simulink model "sampleModel1414"  (R2023a)
settings: Solver=VariableStepAuto  StartTime=0.0  StopTime=10.0  RelTol=1e-3
libraries: hdlsllib x2, simulink x2
settings Model: Creator=user1  LastModifiedBy=user1

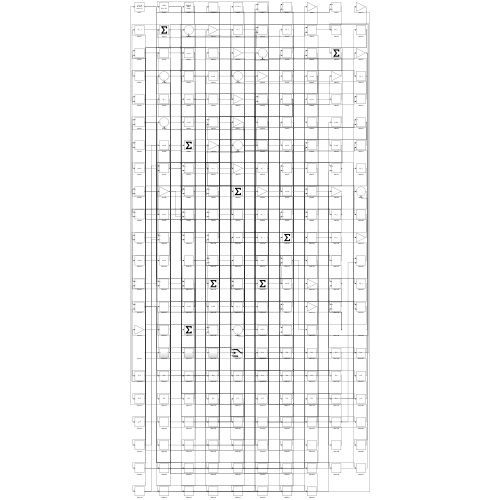
[thumbnail: Simulink's stored preview of the top-level diagram]
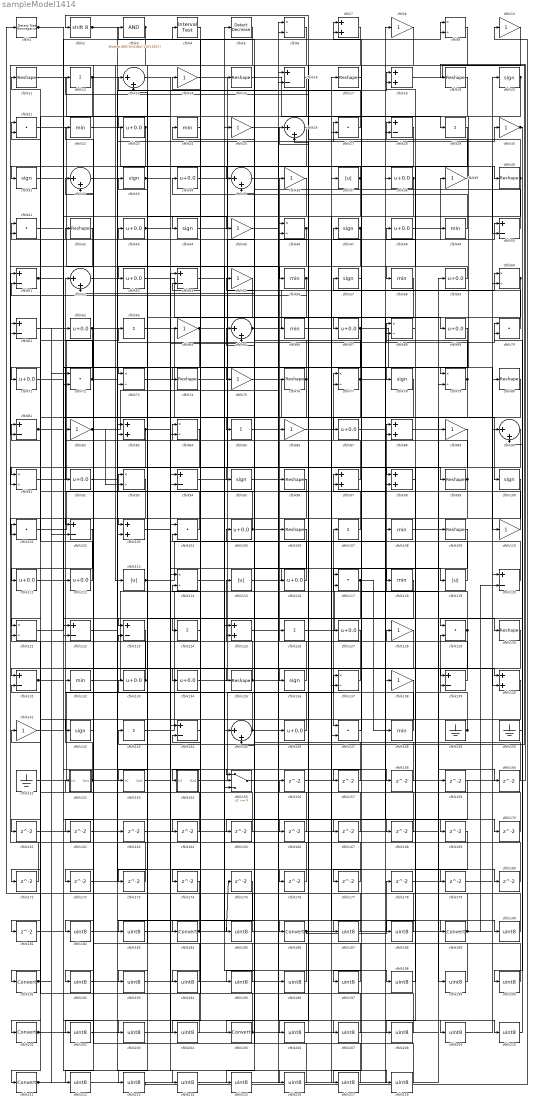
== system sampleModel1414 ==
  cfblk1 : hdlsllib/Logic and Bit Operations/Detect Rise Nonnegative  vinit=0  OutDataTypeStr=boolean
  cfblk{8,10,14,25,30,36,39,45,55,64,75,82,86,89,110,128,138,141} (18 alike) : Gain
  cfblk{20,31,33,44,47,57,78,95,100,136,142} (11 alike) : Signum
  cfblk{21,27,41,70,72,101,104,117,129,147} (10 alike) : DotProduct  OutDataTypeStr=Inherit: Inherit via internal rule
  cfblk{16,28,50..51,54,61,81,94,102,120,122..123,131,139,144} (15 alike) : Sum  Inputs=+-
  cfblk{7,18,83,88,97..98,103,125,140} (9 alike) : Sum
  cfblk{23,34,38,43,48,53,59,62,67,69,71,87,92,105,111..112,116,127,133..134,146} (21 alike) : Bias  Bias=0.0  SaturateOnIntegerOverflow=off
  cfblk{11,15,17,19,40,42,74,76,80,96,99,106,109,130,135} (15 alike) : Reshape
  cfblk{12,29,63,85,107,124,126,143} (8 alike) : Sum  Inputs=+
  cfblk{22,24,49,56,58,66,108,118,132,148} (10 alike) : MinMax
  cfblk{37,113,115,119} (4 alike) : Abs  SaturateOnIntegerOverflow=off
  cfblk{6,9,46,60,68,73,77,79,84,91,93,114,121,137} (14 alike) : Product  Inputs=*/  RndMeth=Zero  SaturateOnIntegerOverflow=on
  cfblk{13,26,32,35,52,65,90,145} (8 alike) : Sum  Inputs=|++
  cfblk149 : Ground
  cfblk150 : Ground
  cfblk151 : Ground
  cfblk152 : Subsystem
      settings: LibrarySourceBlock=|
      | hdlsllib/Ports &
      | Subsystems/Subsystem
  cfblk153 : Subsystem
      settings: LibrarySourceBlock=|
      | hdlsllib/Ports &
      | Subsystems/Subsystem
  cfblk154 : Subsystem
      settings: LibrarySourceBlock=|
      | hdlsllib/Ports &
      | Subsystems/Subsystem
  cfblk155 : Switch  SaturateOnIntegerOverflow=off  InputSameDT=off
  cfblk{156..181} (26 alike) : Delay  SampleTime=1
  cfblk{182..183,185,187..188,190,192..200,202..204,206..210,212..218} (30 alike) : DataTypeConversion  OutDataTypeStr=uint8  SaturateOnIntegerOverflow=off  RndMeth=Floor
  cfblk{184,186,189,191,201,205,211} (7 alike) : DataTypeConversion  SaturateOnIntegerOverflow=off  RndMeth=Floor
  cfblk2 : ArithShift  BitShiftNumber=8
  cfblk3 : simulink/Logic and Bit Operations/Bitwise Operator  logicop=AND  UseBitMask=on  BitMask=bin2dec('11011001')  BitMaskRealWorld=Stored Integer
      settings: LibrarySourceBlock=|
      | hdlsllib/Logic and Bit
      | Operations/Bitwise
      | Operator
  cfblk4 : hdlsllib/Logic and Bit Operations/Interval Test  IntervalClosedRight=on  uplimit=0.5  IntervalClosedLeft=on  lowlimit=-0.5  OutDataTypeStr=boolean
  cfblk5 : simulink/Logic and Bit Operations/Detect Decrease  vinit=0.0  OutDataTypeStr=boolean
      settings: LibrarySourceBlock=|
      | hdlsllib/Logic and Bit
      | Operations/Detect
      | Decrease
  wires:
  cfblk97/1 -> cfblk36/1
  cfblk57/1 -> cfblk103/1
  cfblk53/1 -> cfblk67/1
  cfblk3/1 -> cfblk113/1, cfblk81/2
  cfblk136/1 -> cfblk86/1
  cfblk39/1 -> cfblk2/1
  cfblk20/1 -> cfblk78/1, cfblk71/1
  cfblk145/1 -> cfblk33/1, cfblk49/1
  cfblk98/1 -> cfblk48/1
  cfblk50/1 -> cfblk24/1
  cfblk113/1 -> cfblk38/1, cfblk117/2
  cfblk152/1(Out1) -> cfblk52/1, cfblk155/2
  cfblk107/1 -> cfblk97/1
  cfblk89/1 -> cfblk211/1
  cfblk79/1 -> cfblk28/1, cfblk187/1
  cfblk94/1 -> cfblk60/1
  cfblk34/1 -> cfblk40/1
  cfblk30/1 -> cfblk129/1, cfblk200/1
  cfblk45/1 -> cfblk106/1
  cfblk134/1 -> cfblk50/1
  cfblk148/1 -> cfblk84/1
  cfblk135/1 -> cfblk115/1, cfblk210/1
  cfblk26/1 -> cfblk205/1
  cfblk77/1 -> cfblk41/1, cfblk127/1, cfblk140/1, cfblk161/1
  cfblk63/1 -> cfblk100/1
  cfblk14/1 -> cfblk99/1
  cfblk48/1 -> cfblk39/1
  cfblk124/1 -> cfblk14/1
  cfblk91/1 -> cfblk63/1
  cfblk44/1 -> cfblk27/1
  cfblk129/1 -> cfblk47/1, cfblk139/1
  cfblk76/1 -> cfblk3/1, cfblk103/2
  cfblk27/1 -> cfblk13/1
  cfblk60/1 -> cfblk98/2, cfblk204/1
  cfblk2/1 -> cfblk56/1, cfblk176/1
  cfblk123/1 -> cfblk131/1
  cfblk21/1 -> cfblk125/1
  cfblk149/1 -> cfblk129/2, cfblk68/2, cfblk139/2
  cfblk18/1 -> cfblk143/1
  cfblk151/1 -> cfblk15/1
  cfblk65/1 -> cfblk20/1, cfblk9/1
  cfblk62/1 -> cfblk92/1, cfblk30/1
  cfblk109/1 -> cfblk147/1
  cfblk22/1 -> cfblk50/2
  cfblk75/1 -> cfblk109/1
  cfblk35/1 -> cfblk69/1
  cfblk82/1 -> cfblk76/1, cfblk93/2
  cfblk81/1 -> cfblk122/1, cfblk140/2
  cfblk67/1 -> cfblk110/1, cfblk122/2
  cfblk70/1 -> cfblk7/1
  cfblk68/1 -> cfblk18/1
  cfblk143/1 -> cfblk107/1
  cfblk13/1 -> cfblk45/1
  cfblk133/1 -> cfblk101/1, cfblk93/1
  cfblk154/1(Out1) -> cfblk137/1
  cfblk99/1 -> cfblk22/1, cfblk77/2, cfblk165/1
  cfblk46/1 -> cfblk94/2, cfblk74/1
  cfblk11/1 -> cfblk84/2
  cfblk96/1 -> cfblk101/2
  cfblk132/1 -> cfblk59/1
  cfblk28/1 -> cfblk41/2
  cfblk117/1 -> cfblk153/1(In1), cfblk148/1
  cfblk155/1 -> cfblk19/1
  cfblk131/1 -> cfblk102/2, cfblk207/1, cfblk209/1
  cfblk1/1 -> cfblk44/1, cfblk9/2
  cfblk61/1 -> cfblk123/1
  cfblk150/1 -> cfblk70/1
  cfblk105/1 -> cfblk119/1, cfblk21/2
  cfblk85/1 -> cfblk126/1
  cfblk64/1 -> cfblk25/1, cfblk102/1
  cfblk38/1 -> cfblk95/1, cfblk87/1
  cfblk139/1 -> cfblk82/1
  cfblk115/1 -> cfblk117/1
  cfblk42/1 -> cfblk61/2
  cfblk9/1 -> cfblk35/1
  cfblk37/1 -> cfblk154/1(In1), cfblk31/1
  cfblk126/1 -> cfblk88/1
  cfblk54/1 -> cfblk145/1
  cfblk55/1 -> cfblk73/1
  cfblk49/1 -> cfblk34/1
  cfblk138/1 -> cfblk201/1
  cfblk114/1 -> cfblk186/1
  cfblk121/1 -> cfblk7/2
  cfblk59/1 -> cfblk53/1
  cfblk15/1 -> cfblk29/1
  cfblk12/1 -> cfblk72/2, cfblk180/1
  cfblk104/1 -> cfblk21/1
  cfblk146/1 -> cfblk42/1
  cfblk137/1 -> cfblk136/1
  cfblk29/1 -> cfblk58/1
  cfblk120/1 -> cfblk54/2
  cfblk25/1 -> cfblk116/1
  cfblk56/1 -> cfblk51/2, cfblk134/1
  cfblk147/1 -> cfblk57/1
  cfblk69/1 -> cfblk142/1
  cfblk73/1 -> cfblk146/1
  cfblk116/1 -> cfblk55/1
  cfblk119/1 -> cfblk46/2
  cfblk8/1 -> cfblk23/1
  cfblk4/1 -> cfblk184/1
  cfblk72/1 -> cfblk18/2, cfblk11/1, cfblk98/1
  cfblk40/1 -> cfblk137/2, cfblk12/1
  cfblk47/1 -> cfblk124/1, cfblk155/3, cfblk206/1
  cfblk112/1 -> cfblk81/1
  cfblk51/1 -> cfblk130/1, cfblk75/1, cfblk91/1
  cfblk71/1 -> cfblk112/1
  cfblk43/1 -> cfblk118/1, cfblk155/1
  cfblk86/1 -> cfblk77/1
  cfblk66/1 -> cfblk189/1
  cfblk58/1 -> cfblk135/1
  cfblk101/1 -> cfblk8/1
  cfblk31/1 -> cfblk85/1
  cfblk23/1 -> cfblk121/1, cfblk192/1
  cfblk103/1 -> cfblk70/2
  cfblk122/1 -> cfblk68/1
  cfblk33/1 -> cfblk79/1, cfblk179/1
  cfblk16/1 -> cfblk191/1
  cfblk110/1 -> cfblk97/2
  cfblk19/1 -> cfblk111/1
  cfblk80/1 -> cfblk83/2
  cfblk83/1 -> cfblk65/2, cfblk91/2
  cfblk156/1 -> cfblk27/2
  cfblk78/1 -> cfblk157/1
  cfblk157/1 -> cfblk104/1
  cfblk41/1 -> cfblk158/1
  cfblk158/1 -> cfblk94/1
  cfblk88/1 -> cfblk160/1
  cfblk160/1 -> cfblk52/2
  cfblk161/1 -> cfblk79/2
  cfblk140/1 -> cfblk162/1
  cfblk162/1 -> cfblk54/1
  cfblk92/1 -> cfblk163/1
  cfblk24/1 -> cfblk164/1
  cfblk164/1 -> cfblk123/2
  cfblk165/1 -> cfblk131/2
  cfblk7/1 -> cfblk166/1
  cfblk166/1 -> cfblk65/1
  cfblk111/1 -> cfblk167/1
  cfblk167/1 -> cfblk35/2
  cfblk95/1 -> cfblk168/1
  cfblk168/1 -> cfblk125/2
  cfblk87/1 -> cfblk169/1
  cfblk153/1(Out1) -> cfblk170/1
  cfblk170/1 -> cfblk145/2
  cfblk84/1 -> cfblk171/1
  cfblk171/1 -> cfblk61/1
  cfblk93/1 -> cfblk172/1
  cfblk172/1 -> cfblk73/2
  cfblk130/1 -> cfblk173/1
  cfblk173/1 -> cfblk51/1
  cfblk118/1 -> cfblk174/1
  cfblk174/1 -> cfblk1/1
  cfblk176/1 -> cfblk13/2
  cfblk17/1 -> cfblk177/1
  cfblk177/1 -> cfblk83/1
  cfblk178/1 -> cfblk120/1
  cfblk179/1 -> cfblk60/2
  cfblk180/1 -> cfblk46/1
  cfblk102/1 -> cfblk181/1
  cfblk5/1 -> cfblk182/1
  cfblk182/1 -> cfblk37/1
  cfblk36/1 -> cfblk183/1
  cfblk183/1 -> cfblk5/1
  cfblk184/1 -> cfblk175/1, cfblk43/1
  cfblk100/1 -> cfblk185/1
  cfblk185/1 -> cfblk4/1
  cfblk186/1 -> cfblk178/1, cfblk80/1
  cfblk187/1 -> cfblk114/1
  cfblk169/1 -> cfblk188/1
  cfblk188/1 -> cfblk114/2
  cfblk189/1 -> cfblk156/1, cfblk120/2
  cfblk52/1 -> cfblk190/1
  cfblk190/1 -> cfblk66/1
  cfblk191/1 -> cfblk121/2, cfblk72/1
  cfblk192/1 -> cfblk16/1
  cfblk175/1 -> cfblk193/1
  cfblk193/1 -> cfblk16/2
  cfblk144/1 -> cfblk194/1
  cfblk194/1 -> cfblk152/1(In1)
  cfblk159/1 -> cfblk195/1
  cfblk195/1 -> cfblk144/1
  cfblk125/1 -> cfblk196/1
  cfblk196/1 -> cfblk144/2
  cfblk128/1 -> cfblk197/1
  cfblk197/1 -> cfblk133/1
  cfblk74/1 -> cfblk198/1
  cfblk198/1 -> cfblk128/1
  cfblk108/1 -> cfblk199/1
  cfblk199/1 -> cfblk96/1
  cfblk200/1 -> cfblk108/1
  cfblk201/1 -> cfblk159/1, cfblk88/2
  cfblk127/1 -> cfblk202/1
  cfblk202/1 -> cfblk138/1
  cfblk141/1 -> cfblk203/1
  cfblk203/1 -> cfblk64/1
  cfblk204/1 -> cfblk141/1
  cfblk205/1 -> cfblk147/2, cfblk132/1
  cfblk206/1 -> cfblk26/1
  cfblk207/1 -> cfblk26/2
  cfblk90/1 -> cfblk208/1
  cfblk208/1 -> cfblk104/2
  cfblk209/1 -> cfblk90/1
  cfblk210/1 -> cfblk90/2
  cfblk211/1 -> cfblk28/2, cfblk17/1, cfblk62/1
  cfblk142/1 -> cfblk212/1
  cfblk212/1 -> cfblk89/1
  cfblk6/1 -> cfblk213/1
  cfblk213/1 -> cfblk10/1
  cfblk181/1 -> cfblk214/1
  cfblk214/1 -> cfblk6/1
  cfblk106/1 -> cfblk215/1
  cfblk215/1 -> cfblk6/2
  cfblk32/1 -> cfblk216/1
  cfblk216/1 -> cfblk105/1
  cfblk10/1 -> cfblk217/1
  cfblk217/1 -> cfblk32/1
  cfblk163/1 -> cfblk218/1
  cfblk218/1 -> cfblk32/2

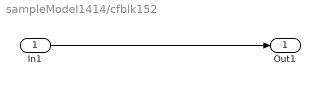
== system sampleModel1414/cfblk152 ==
  In1 : Inport
  Out1 : Outport
  wires:
  In1/1 -> Out1/1

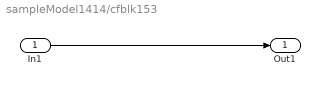
== system sampleModel1414/cfblk153 ==
  In1 : Inport
  Out1 : Outport
  wires:
  In1/1 -> Out1/1

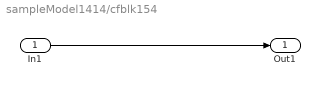
== system sampleModel1414/cfblk154 ==
  In1 : Inport
  Out1 : Outport
  wires:
  In1/1 -> Out1/1
